simulink model "trainCOMPLETE_discrete_firction_2D"  (Simulink 7.8)
settings: Solver=FixedStepDiscrete  StartTime=0.0  StopTime=10.0  FixedStep=Delta_t  RelTol=1e-3
values from neighbouring files (symbols this model uses):
  q = [xWAG;zWAG;bWAG;zRBOG;bRBOG;zFBOG;bFBOG;zRWHSF;bRWHSF;zRWHSR;bRWHSR;zFWHSF;bFWHSF;zFWHSR;bFWHSR;bRAXBFR;bRAXBRR;bFAXBFR;bFAXBRR;xRMOTF;zRMOTF;bRMOTF;xRMOTR;zRMOTR;bRMOTR;bRROTF;bRROTR;RthetaWRF;RthetaWRR;RxRRF;RxRRR;FthetaWRF;FthetaWRR;FxRRF;FxRRR;]    [environment.m]
undefined symbols (not defined in the file or in its folder): Delta_t
settings Model: Creator=imac  LastModifiedBy=aitor
settings DebuggingCC: FcnCallInpInsideContextMsg=Use local settings

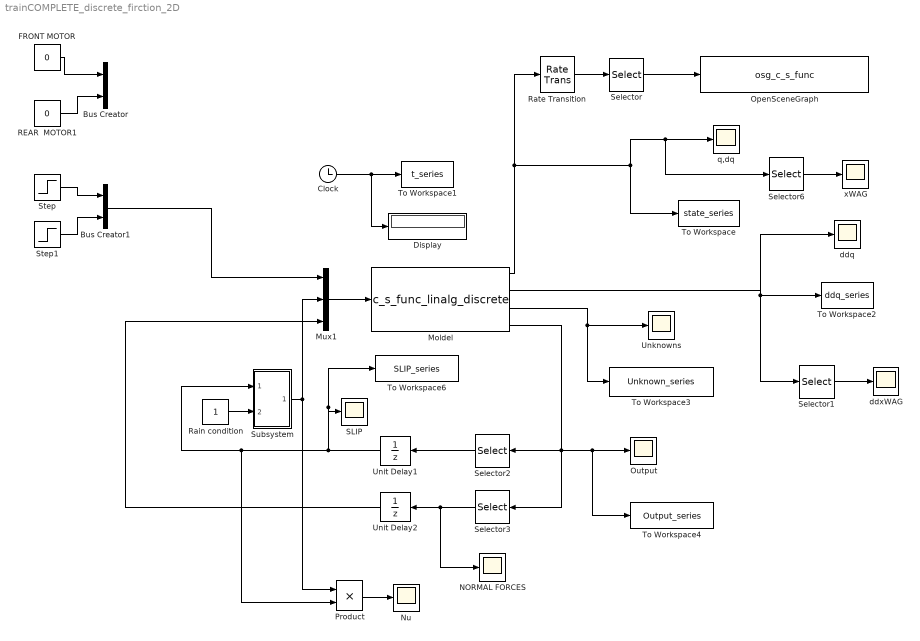
== system trainCOMPLETE_discrete_firction_2D ==
  Bus Creator : BusCreator  Inputs=2
  Bus Creator1 : BusCreator  Inputs=2
  Clock : Clock
  Display : Display
  FRONT MOTOR : Constant  Value=0
  Moldel : S-Function  FunctionName=c_s_func_linalg_discrete  Parameters=q dq param Delta_t  EnableBusSupport=off
      mask Type: S-function: mycsfunc
      mask Description: This is a S-function that does the continuous state space system.
      mask Display: disp('[M , Phi_q''] [ddq]\n[Phi_q , 0] [lambda]\n=\n [Q ] \n   [gamma] ');
  Mux1 : Mux  Inputs=3
  NORMAL FORCES : Scope
      settings: TimeRange=10  YMin=40000  YMax=145000  SaveName=Normal  DataFormat=Array  SampleInput=on  SampleTime=Delta_t
  Nu : Scope
      settings: TimeRange=10  YMin=-4.33681e-18  YMax=0.0575  SaveName=Nu  DataFormat=Array  SampleInput=on  SampleTime=Delta_t
  OpenSceneGraph : S-Function  FunctionName=osg_c_s_func  EnableBusSupport=off
  Output : Scope
      settings: YMin=0  YMax=750000  SaveName=ScopeData5  SampleInput=on  SampleTime=Delta_t
  Product : Product  RndMeth=Zero
  REAR  MOTOR1 : Constant  Value=0
  Rain condition : Constant
  Rate Transition : RateTransition  OutPortSampleTime=0.01
  SLIP : Scope
      settings: TimeRange=10  YMin=1.04083e-17  YMax=0.22  SaveName=SLIP  DataFormat=Array  SampleInput=on
  Selector : Selector  InputPortWidth=2*length(q)  IndexOptions=Index vector (dialog)  Indices=1:1:length(q)  OutputSizes=1
  Selector1 : Selector  InputPortWidth=length(q)  IndexOptions=Index vector (dialog)  Indices=1  OutputSizes=1
  Selector2 : Selector  InputPortWidth=8  IndexOptions=Index vector (dialog)  Indices=1:1:4  OutputSizes=1
  Selector3 : Selector  InputPortWidth=8  IndexOptions=Index vector (dialog)  Indices=5:1:8  OutputSizes=1
  Selector6 : Selector  InputPortWidth=2*length(q)  IndexOptions=Index vector (dialog)  Indices=1  OutputSizes=1
  Step : Step  Time=3  After=-1700  SampleTime=0
  Step1 : Step  Time=3  After=-1700  SampleTime=0
  Subsystem : Subsystem
  To Workspace : ToWorkspace  VariableName=state_series  SampleTime=-1  SaveFormat=Array
  To Workspace1 : ToWorkspace  VariableName=t_series  SampleTime=-1  SaveFormat=Array
  To Workspace2 : ToWorkspace  VariableName=ddq_series  SampleTime=-1  SaveFormat=Array
  To Workspace3 : ToWorkspace  VariableName=Unknown_series  SampleTime=-1  SaveFormat=Array
  To Workspace4 : ToWorkspace  VariableName=Output_series  SampleTime=Delta_t  SaveFormat=Array
  To Workspace6 : ToWorkspace  VariableName=SLIP_series  SampleTime=-1  SaveFormat=Array
  Unit Delay1 : UnitDelay  SampleTime=-1
  Unit Delay2 : UnitDelay  SampleTime=-1
  Unknowns : Scope
      settings: YMin=0  YMax=140000  SaveName=ScopeData2  SampleInput=on  SampleTime=Delta_t
  ddq : Scope
      settings: YMin=-1050  YMax=50  SampleInput=on
  ddxWAG : Scope
      settings: TimeRange=10  YMin=0.031  YMax=0.054  SaveName=ddxWAG  DataFormat=Array
  q,dq : Scope
      settings: YMin=-0.03  YMax=0.17  SampleInput=on
  xWAG : Scope
      settings: TimeRange=10  YMin=4.65  YMax=5.75  SaveName=xWAG  DataFormat=Array
  wires:
  Clock/1 -> To Workspace1/1, Display/1
  Moldel/1 -> To Workspace/1, q,dq/1, Selector6/1, Rate Transition/1
  Moldel/2 -> ddq/1, To Workspace2/1, Selector1/1
  Moldel/3 -> Unknowns/1, To Workspace3/1
  Unit Delay1/1 -> To Workspace6/1, SLIP/1, Subsystem/1(In1), Product/2
  Mux1/1 -> Moldel/1
  Moldel/4 -> To Workspace4/1, Output/1, Selector2/1, Selector3/1
  Selector6/1 -> xWAG/1
  Selector/1 -> OpenSceneGraph/1
  Rate Transition/1 -> Selector/1
  Selector2/1 -> Unit Delay1/1
  Selector3/1 -> Unit Delay2/1, NORMAL FORCES/1
  Rain condition/1 -> Subsystem/2(In2)
  FRONT MOTOR/1 -> Bus Creator/1
  REAR  MOTOR1/1 -> Bus Creator/2
  Unit Delay2/1 -> Mux1/3
  Subsystem/1(Out1) -> Mux1/2, Product/1
  Step/1 -> Bus Creator1/1
  Step1/1 -> Bus Creator1/2
  Selector1/1 -> ddxWAG/1
  Product/1 -> Nu/1
  Bus Creator1/1 -> Mux1/1

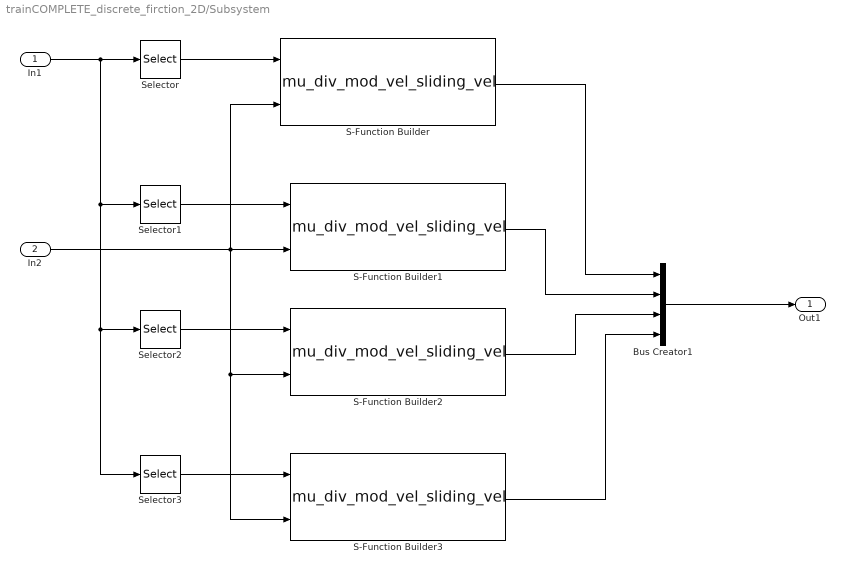
== system trainCOMPLETE_discrete_firction_2D/Subsystem ==
  In1 : Inport
  In2 : Inport  Port=2
  Bus Creator1 : BusCreator
  S-Function Builder : S-Function  InitFcn=try, set_param(gcb,'FunctionName','mu_div_mod_vel_sliding_vel'), end  FunctionName=mu_div_mod_vel_sliding_vel  SFunctionModules=mu_div_mod_vel_sliding_vel_wrapper  WizardData=DataTag0  EnableBusSupport=off  mask(S-Function Builder){}
      mask help: Simulink:masks:SFunctionBuilder_MD
      mask init:
      | val = [[.9  0.75 0.75 1 1 .9 .9 1]',[1 1 0.75 0.75 .9 .9 1 .9]'];try , sys = get_param(gcb,'SfunBuilderFcnName');if isempty(sys), sys = get_param(gcb,'FunctionName'); end,catch, sys = get_param(gcb,'FunctionName'); end
      settings: CopyFcn=set_param(gcbh,'LinkStatus','none')  PreSaveFcn=try, set_param(gcb,'FunctionName','mu_div_mod_vel_sliding_vel'), end  OpenFcn=sfunctionwizard(gcbh)
      mask Display: plot(val(:,1),val(:,2)),disp(sys), port_label('input',1,'u0'), port_label('input',2,'u1'), port_label('output',1,'y0')
  S-Function Builder1 : S-Function  InitFcn=try, set_param(gcb,'FunctionName','mu_div_mod_vel_sliding_vel'), end  FunctionName=mu_div_mod_vel_sliding_vel  SFunctionModules=mu_div_mod_vel_sliding_vel_wrapper  WizardData=DataTag1  EnableBusSupport=off  mask(S-Function Builder){}
      mask help: Simulink:masks:SFunctionBuilder_MD
      mask init: same as trainCOMPLETE_discrete_firction_2D/Subsystem/S-Function Builder
      settings: CopyFcn=set_param(gcbh,'LinkStatus','none')  PreSaveFcn=try, set_param(gcb,'FunctionName','mu_div_mod_vel_sliding_vel'), end  OpenFcn=sfunctionwizard(gcbh)
      mask Display: plot(val(:,1),val(:,2)),disp(sys), port_label('input',1,'u0'), port_label('input',2,'u1'), port_label('output',1,'y0')
  S-Function Builder2 : S-Function  InitFcn=try, set_param(gcb,'FunctionName','mu_div_mod_vel_sliding_vel'), end  FunctionName=mu_div_mod_vel_sliding_vel  SFunctionModules=mu_div_mod_vel_sliding_vel_wrapper  WizardData=DataTag2  EnableBusSupport=off  mask(S-Function Builder){}
      mask help: Simulink:masks:SFunctionBuilder_MD
      mask init: same as trainCOMPLETE_discrete_firction_2D/Subsystem/S-Function Builder
      settings: CopyFcn=set_param(gcbh,'LinkStatus','none')  PreSaveFcn=try, set_param(gcb,'FunctionName','mu_div_mod_vel_sliding_vel'), end  OpenFcn=sfunctionwizard(gcbh)
      mask Display: plot(val(:,1),val(:,2)),disp(sys), port_label('input',1,'u0'), port_label('input',2,'u1'), port_label('output',1,'y0')
  S-Function Builder3 : S-Function  InitFcn=try, set_param(gcb,'FunctionName','mu_div_mod_vel_sliding_vel'), end  FunctionName=mu_div_mod_vel_sliding_vel  SFunctionModules=mu_div_mod_vel_sliding_vel_wrapper  WizardData=DataTag3  EnableBusSupport=off  mask(S-Function Builder){}
      mask help: Simulink:masks:SFunctionBuilder_MD
      mask init: same as trainCOMPLETE_discrete_firction_2D/Subsystem/S-Function Builder
      settings: CopyFcn=set_param(gcbh,'LinkStatus','none')  PreSaveFcn=try, set_param(gcb,'FunctionName','mu_div_mod_vel_sliding_vel'), end  OpenFcn=sfunctionwizard(gcbh)
      mask Display: plot(val(:,1),val(:,2)),disp(sys), port_label('input',1,'u0'), port_label('input',2,'u1'), port_label('output',1,'y0')
  Selector : Selector  InputPortWidth=4  IndexOptions=Index vector (dialog)  Indices=1  OutputSizes=1
  Selector1 : Selector  InputPortWidth=4  IndexOptions=Index vector (dialog)  Indices=2  OutputSizes=1
  Selector2 : Selector  InputPortWidth=4  IndexOptions=Index vector (dialog)  Indices=3  OutputSizes=1
  Selector3 : Selector  InputPortWidth=4  IndexOptions=Index vector (dialog)  Indices=4  OutputSizes=1
  Out1 : Outport
  wires:
  S-Function Builder1/1 -> Bus Creator1/2
  Selector1/1 -> S-Function Builder1/1
  Selector/1 -> S-Function Builder/1
  In1/1 -> Selector/1, Selector1/1, Selector2/1, Selector3/1
  S-Function Builder/1 -> Bus Creator1/1
  In2/1 -> S-Function Builder/2, S-Function Builder2/2, S-Function Builder3/2, S-Function Builder1/2
  S-Function Builder2/1 -> Bus Creator1/3
  S-Function Builder3/1 -> Bus Creator1/4
  Selector2/1 -> S-Function Builder2/1
  Selector3/1 -> S-Function Builder3/1
  Bus Creator1/1 -> Out1/1
